simulink model "ThreeDOFHeli"  (R2022b)
settings: Solver=ode45  StartTime=0.0  StopTime=inf  RelTol=1e-3  EnableMultiTasking=on
InitFcn:
  | ThreeDOFHeli_Setup
libraries: jMPClib x2, vrlib x1, simulink x1
settings Model: Creator=Jonathan Currie  LastModifiedBy=Jonathan Currie
settings SolverCC: AlgebraicLoopSolver=TrustRegion
settings DataIOCC: LimitDataPoints=on  SaveFormat=Array  SignalLoggingSaveFormat=ModelDataLogs  ReturnWorkspaceOutputs=off
settings OptimizationCC: ExpressionDepthLimit=2147483647  LifeSpan=inf
settings DebuggingCC: UnderspecifiedInitializationDetection=Classic  MergeDetectMultiDrivingBlocksExec=none  SolverPrmCheckMsg=warning  FcnCallInpInsideContextMsg=warning  UnconnectedInputMsg=warning  UnconnectedOutputMsg=warning  UnconnectedLineMsg=warning  StateNameClashWarn=warning  SFUnexpectedBacktrackingDiag=warning  SFNoUnconditionalDefaultTransitionDiag=warning  SFExecutionAtInitializationDiag=none  SFMachineParentedDataDiag=warning  ArithmeticOperatorsInVariantConditions=warning
settings HardwareCC: ProdBitPerPointer=32  ProdBitPerSizeT=32  ProdBitPerPtrDiffT=32  ProdLargestAtomicFloat=None  ProdIntDivRoundTo=Undefined  ProdEndianess=Unspecified  ProdWordSize=32  ProdHWDeviceType=32-bit Generic
settings ModelReferenceCC: PropagateSignalLabelsOutOfModel=off
settings SFSimCC: SimUseLocalCustomCode=off  CustomCodeUndefinedFunction=UseInterfaceOnly
settings RTWCC: RTWUseLocalCustomCode=off
settings CodeAppCC: StateflowObjectComments=on
settings GRTTargetCC: TargetLangStandard=C89/C90 (ANSI)  CombineOutputUpdateFcns=off  GRTInterface=on
settings ConfigComp: CovMetricSettings=dw  CovSaveCumulativeToWorkspaceVar=on  CovSaveSingleToWorkspaceVar=on  CovExternalEMLEnable=off

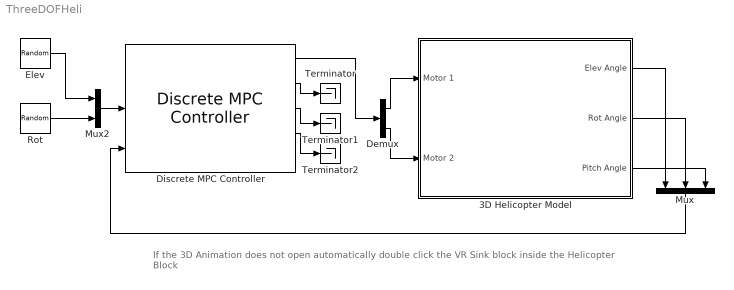
== system ThreeDOFHeli ==
  note: If the 3D Animation does not open automatically double click the VR Sink block inside the Helicopter Block
  3D Helicopter Model : Subsystem
      mask Display:
      | image(imread('Images/3DOFHeliblock.png'))
      | port_label('input', 1, 'V1')
      | port_label('input', 2, 'V2')
      | port_label('output', 1, 'Elev')
      | port_label('output', 2, 'Rot')
      | port_label('output', 3, 'Pitch')
  Demux : Demux  Outputs=2
  Discrete MPC Controller : jMPClib/MPC Blocks/Discrete MPC Controller  SIMJMPC=MPC1
      settings: SourceProductName=JMPC Toolbox
  Elev : RandomNumber  Variance=0.05  Seed=1  SampleTime=20
  Mux : Mux  Inputs=3
  Mux2 : Mux  Inputs=2
  Rot : RandomNumber  Variance=2  Seed=42452  SampleTime=30
  Terminator : Terminator
  Terminator1 : Terminator
  Terminator2 : Terminator
  wires:
  Discrete MPC Controller/1 -> Demux/1
  Mux2/1 -> Discrete MPC Controller/2
  Demux/1 -> 3D Helicopter Model/1(Motor 1)
  Demux/2 -> 3D Helicopter Model/2(Motor 2)
  3D Helicopter Model/1(Elev Angle) -> Mux/1
  3D Helicopter Model/2(Rot Angle) -> Mux/2
  3D Helicopter Model/3(Pitch Angle) -> Mux/3
  Mux/1 -> Discrete MPC Controller/3
  Rot/1 -> Mux2/2
  Elev/1 -> Mux2/1
  Discrete MPC Controller/2 -> Terminator/1
  Discrete MPC Controller/4 -> Terminator2/1
  Discrete MPC Controller/3 -> Terminator1/1

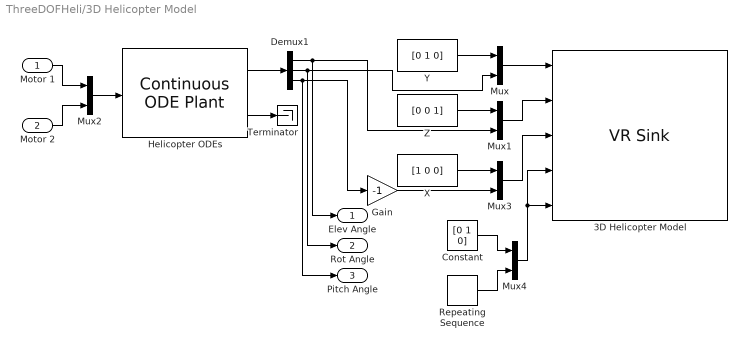
== system ThreeDOFHeli/3D Helicopter Model ==
  Motor 1 : Inport
  Motor 2 : Inport  Port=2
  3D Helicopter Model : vrlib/VR Sink  InstantiateOnLoad=on  SampleTime=0.1  ViewEnable=on  RemoteChange=off  RemoteView=on  FieldsWritten=HelicopterRot.rotation.4.1.1.double#HelicopterElev.rotation.4.1.1.double#HelicopterPitch.rotation.4.1.1.double#Rotor1.rotation.4.1.1.double#Rotor2.rotation.4.1.1.double  WorldFileName=VRML Files\3DOFHeli.wrl  WorldDescription=3DOF Helicopter  AutoView=on  VideoDimensions=[]  AllowVariableSize=off
  Constant : Constant  Value=[0 1 0]
  Demux1 : Demux  Outputs=3
  Gain : Gain  Gain=-1
  Helicopter ODEs : jMPClib/MPC Blocks/Continuous ODE Plant  jNLObj=Plant
      settings: SourceProductName=JMPC Toolbox
  Mux{,1..4} (5 alike) : Mux  Inputs=2
  Repeating Sequence : simulink/Sources/Repeating Sequence  rep_seq_t=0:15  rep_seq_y=linspace(0,20*pi,16)
  Terminator : Terminator
  X : Constant  Value=[1 0 0]
  Y : Constant  Value=[0 1 0]
  Z : Constant  Value=[0 0 1]
  Elev Angle : Outport
  Rot Angle : Outport  Port=2
  Pitch Angle : Outport  Port=3
  wires:
  Z/1 -> Mux1/1
  X/1 -> Mux3/1
  Y/1 -> Mux/1
  Demux1/1 -> Mux1/2, Elev Angle/1
  Demux1/3 -> Pitch Angle/1, Gain/1
  Mux2/1 -> Helicopter ODEs/1
  Motor 1/1 -> Mux2/1
  Motor 2/1 -> Mux2/2
  Helicopter ODEs/1 -> Demux1/1
  Demux1/2 -> Mux/2, Rot Angle/1
  Helicopter ODEs/2 -> Terminator/1
  Mux/1 -> 3D Helicopter Model/1
  Mux1/1 -> 3D Helicopter Model/2
  Mux3/1 -> 3D Helicopter Model/3
  Constant/1 -> Mux4/1
  Repeating Sequence/1 -> Mux4/2
  Mux4/1 -> 3D Helicopter Model/5, 3D Helicopter Model/4
  Gain/1 -> Mux3/2
